simulink model "TITO_OCD_DE_2011"  (Simulink 7.7)
settings: Solver=ode4  SolverMode=SingleTasking  StartTime=0.0  StopTime=100  RelTol=1e-3  AbsTol=1e-6
libraries: simulink x40, stcsl_std x2
settings Model: Creator=chalupa  LastModifiedBy=NICHOLAS ANG
settings DataIOCC: LimitDataPoints=off  SignalLoggingSaveFormat=Dataset  SaveOutput=off  SaveTime=off
settings OptimizationCC: BlockReduction=off  BooleanDataType=off  ExpressionDepthLimit=128  InitFltsAndDblsToZero=on
settings DebuggingCC: SaveWithParameterizedLinksMsg=none  SignalResolutionControl=TryResolveAllWithWarning  SolverPrmCheckMsg=none  MultiTaskDSMMsg=warning  MultiTaskCondExecSysMsg=none  FcnCallInpInsideContextMsg=Enable All  StateNameClashWarn=none
settings HardwareCC: ProdBitPerPointer=64  ProdLargestAtomicFloat=Float  ProdIntDivRoundTo=Zero  ProdEndianess=LittleEndian  ProdHWDeviceType=Specified  TargetUnknown=on
settings RTWCC: TemplateMakefile=grt_msvc.tmf
settings CodeAppCC: CustomSymbolStrType=$N$R$M_T
settings GRTTargetCC: TargetFcnLib=ansi_tfl_tmw.mat  TargetFunctionLibrary=C89/C90 (ANSI)  GeneratePreprocessorConditionals=Use local settings

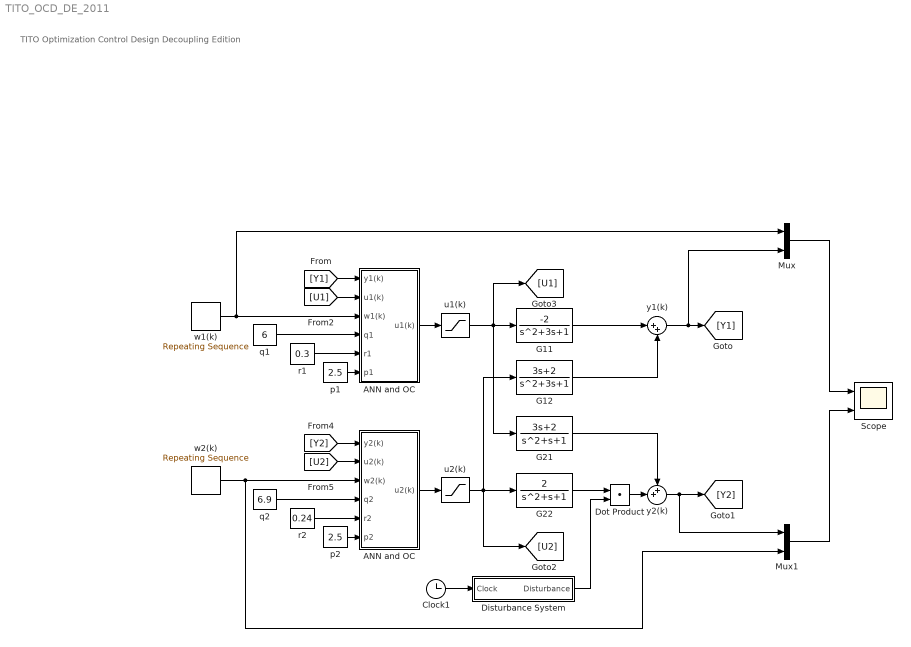
== system TITO_OCD_DE_2011 ==
  note: TITO Optimization Control Design Decoupling Edition
  " ANN and OC " : Subsystem
  ANN and OC : Subsystem
  Clock1 : Clock
  Disturbance System : Subsystem
  Dot Product : DotProduct  InputSameDT=on  OutDataTypeStr=Inherit: Inherit via internal rule
  G11 : TransferFcn  Numerator=[-2]  Denominator=[1 3 1]
  G12 : TransferFcn  Numerator=[3 2]  Denominator=[1 3 1]
  G21 : TransferFcn  Numerator=[3 2]  Denominator=[1 1 1]
  G22 : TransferFcn  Numerator=[2]  Denominator=[1 1 1]
  Mux : Mux  Inputs=2
  Mux1 : Mux  Inputs=2
  "Scope  " : Scope  NumInputPorts=2
      settings: TimeRange=auto  MaxDataPoints=5000  SaveToWorkspace=off  SaveName=ScopeData2  YMin=-1.079~-5  YMax=2.42451~5  SampleTime=-1
  p1 : Constant  Value=2.5
  p2 : Constant  Value=2.5
  q1 : Constant  Value=6
  q2 : Constant  Value=6.9
  r1 : Constant  Value=0.3
  r2 : Constant  Value=0.24
  u1(k) : Saturate  UpperLimit=1  LowerLimit=-1
  u2(k) : Saturate  UpperLimit=1  LowerLimit=-1
  w1(k) : simulink/Sources/Repeating Sequence  rep_seq_t=20*[0 0.4999 0.5 1.4999]  rep_seq_y=[1 1 2 2]
  w2(k) : simulink/Sources/Repeating Sequence  rep_seq_t=20*[0 0.9999 1.0 1.4999]  rep_seq_y=0.52*[1 1 2 2]
  y1(k) : Sum  Inputs=|++
  y2(k) : Sum  Inputs=++|
  wires:
  G11/1 -> y1(k)/1
  G21/1 -> y2(k)/1
  q1/1 -> ANN and OC/4(q1)
  r1/1 -> ANN and OC/5(r1)
  p1/1 -> ANN and OC/6(p1)
  q2/1 -> " ANN and OC "/4(q2)
  r2/1 -> " ANN and OC "/5(r2)
  p2/1 -> " ANN and OC "/6(p2)
  w1(k)/1 -> Mux/1, ANN and OC/3(w1(k))
  w2(k)/1 -> Mux1/2, " ANN and OC "/3(w2(k))
  y2(k)/1 -> Mux1/1, [Y2]
  G12/1 -> y1(k)/2
  [Y1] -> ANN and OC/1(y1(k))
  [U1] -> ANN and OC/2(u1(k))
  " ANN and OC "/1(" u2(k)") -> u2(k)/1
  [U2] -> " ANN and OC "/2(u2(k))
  [Y2] -> " ANN and OC "/1(y2(k))
  ANN and OC/1(" u1(k)") -> u1(k)/1
  u1(k)/1 -> [U1], G21/1, G11/1
  u2(k)/1 -> [U2], G12/1, G22/1
  Clock1/1 -> Disturbance System/1(Clock)
  G22/1 -> Dot Product/1
  Disturbance System/1(Disturbance) -> Dot Product/2
  Dot Product/1 -> y2(k)/2
  Mux/1 -> "Scope  "/1
  Mux1/1 -> "Scope  "/2
  y1(k)/1 -> Mux/2, [Y1]

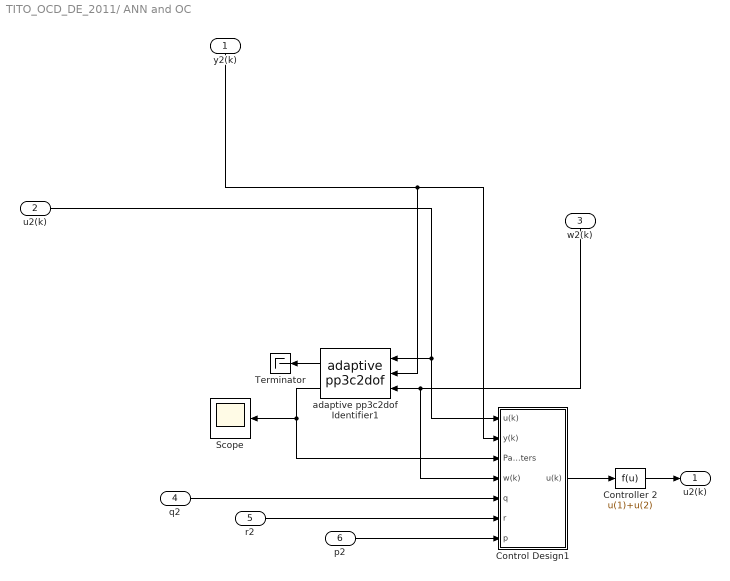
== system TITO_OCD_DE_2011/ ANN and OC  ==
  y2(k) : Inport
  u2(k) : Inport  Port=2
  w2(k) : Inport  Port=3
  q2 : Inport  Port=4
  r2 : Inport  Port=5
  p2 : Inport  Port=6
  " Controller 2 " : Fcn  Expr=u(1)+u(2)
  Control Design1 : Subsystem
  "Scope  " : Scope
      settings: TimeRange=auto  MaxDataPoints=5000  SaveToWorkspace=off  SaveName=ScopeData2  YMin=-1.20758  YMax=0.87657  SampleTime=-1
  Terminator : Terminator
  adaptive pp3c2dof Identifier1 : stcsl_std/Other simple adaptive controllers  using 3rd order models (3)/adaptive pp3c2dof  T0=0.1  ID_type=Least squares method (LSM)  Theta0=[0.1;0.2;0.3;0.4;0.5;0.6]  C0=1e9*eye(6)  phi0=1  lambda0=0.001  rho=0.99  nu0=1e-6  xi=1  omega=1
  " u2(k)" : Outport
  wires:
  y2(k)/1 -> Control Design1/2("y(k)  "), adaptive pp3c2dof Identifier1/2
  u2(k)/1 -> Control Design1/1("u(k)  "), adaptive pp3c2dof Identifier1/1
  adaptive pp3c2dof Identifier1/2 -> "Scope  "/1, Control Design1/3(Parameters)
  p2/1 -> Control Design1/7(p)
  r2/1 -> Control Design1/6(r)
  q2/1 -> Control Design1/5(q)
  Control Design1/1("u(k) ") -> " Controller 2 "/1
  w2(k)/1 -> Control Design1/4(w(k)), adaptive pp3c2dof Identifier1/3
  adaptive pp3c2dof Identifier1/1 -> Terminator/1
  " Controller 2 "/1 -> " u2(k)"/1

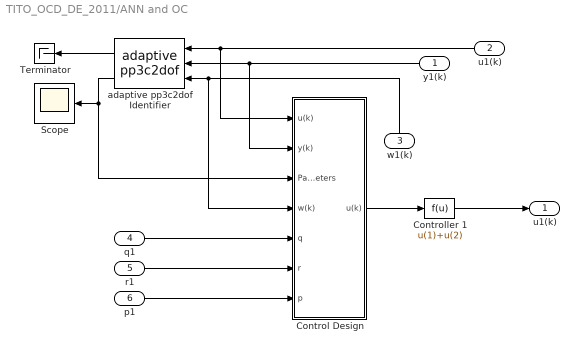
== system TITO_OCD_DE_2011/ANN and OC ==
  y1(k) : Inport
  u1(k) : Inport  Port=2
  w1(k) : Inport  Port=3
  q1 : Inport  Port=4
  r1 : Inport  Port=5
  p1 : Inport  Port=6
  " Controller 1 " : Fcn  Expr=u(1)+u(2)
  Control Design : Subsystem
  "Scope  " : Scope
      settings: TimeRange=auto  MaxDataPoints=5000  SaveToWorkspace=off  YMin=-0.80778  YMax=1.95673  SampleTime=-1
  Terminator : Terminator
  adaptive pp3c2dof Identifier : stcsl_std/Other simple adaptive controllers  using 3rd order models (3)/adaptive pp3c2dof  T0=0.1  ID_type=Least squares method (LSM)  Theta0=[0.1;0.2;0.3;0.4;0.5;0.6]  C0=1e9*eye(6)  phi0=1  lambda0=0.001  rho=0.99  nu0=1e-6  xi=1  omega=1
  " u1(k)" : Outport
  wires:
  u1(k)/1 -> Control Design/1("u(k)  "), adaptive pp3c2dof Identifier/1
  y1(k)/1 -> Control Design/2("y(k)  "), adaptive pp3c2dof Identifier/2
  adaptive pp3c2dof Identifier/2 -> "Scope  "/1, Control Design/3(Parameters)
  p1/1 -> Control Design/7(p)
  q1/1 -> Control Design/5(q)
  r1/1 -> Control Design/6(r)
  w1(k)/1 -> Control Design/4(w(k)), adaptive pp3c2dof Identifier/3
  adaptive pp3c2dof Identifier/1 -> Terminator/1
  Control Design/1("u(k) ") -> " Controller 1 "/1
  " Controller 1 "/1 -> " u1(k)"/1

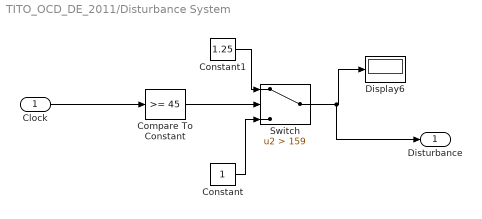
== system TITO_OCD_DE_2011/Disturbance System ==
  Clock : Inport
  Compare To Constant : simulink/Logic and Bit Operations/Compare To Constant  relop=>=  const=45  LogicOutDataTypeMode=boolean
  Constant : Constant
  Constant1 : Constant  Value=1.25
  Display6 : Display
  Switch : Switch  Criteria=u2 > Threshold  Threshold=159
  Disturbance : Outport
  wires:
  Compare To Constant/1 -> Switch/2
  Constant/1 -> Switch/3
  Constant1/1 -> Switch/1
  Switch/1 -> Disturbance/1, Display6/1
  Clock/1 -> Compare To Constant/1

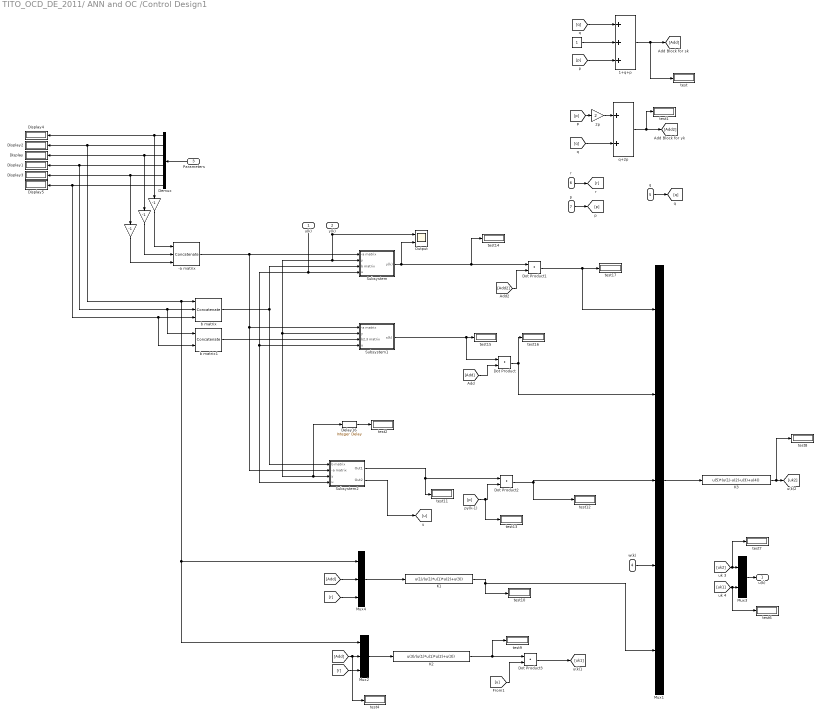
== system TITO_OCD_DE_2011/ ANN and OC /Control Design1 ==
  "u(k)  " : Inport
  "y(k)  " : Inport  Port=2
  Parameters : Inport  Port=3
  w(k) : Inport  Port=4
  q : Inport  Port=5
  r : Inport  Port=6
  p : Inport  Port=7
  " " : Gain  Gain=-1
  "   " : Gain  Gain=-1
  "    " : Gain  Gain=-1
  "      " : Constant
  -a matrix : Concatenate  NumInputs=3  Mode=Multidimensional array  ConcatenateDimension=2
  1+q+p : Sum  Inputs=+++
  2p : Gain  Gain=2
  Delay16 : simulink/Discrete/Integer Delay  NumDelays=1  vinit=0.0  samptime=-1
  Demux : Demux  Outputs=6
  Display{,1..5} (6 alike) : Display
  Dot Product{,1..3} (4 alike) : DotProduct  InputSameDT=on  OutDataTypeStr=Inherit: Inherit via internal rule
  K1 : Fcn  Expr=u(1)/(u(1)*u(1)*u(2)+u(3))
  K2 : Fcn  Expr=u(3)/(u(1)*u(1)*u(2)+u(3))
  K3 : Fcn  Expr=u(5)*(u(1)-u(2)-u(3)+u(4))
  Mux1 : Mux  Inputs=5
  Mux2 : Mux  Inputs=3
  Mux3 : Mux  Inputs=2
  Mux4 : Mux  Inputs=3
  Output : Scope  NumInputPorts=2
      settings: TimeRange=auto  MaxDataPoints=5000  SaveName=ScopeData222  YMin=-1.36833~-5  YMax=12.31494~5  SampleTime=-1
  Subsystem : Subsystem
  Subsystem1 : Subsystem
  Subsystem2 : Subsystem
  b matrix : Concatenate  NumInputs=3  Mode=Multidimensional array  ConcatenateDimension=2
  b matrix1 : Concatenate  Mode=Multidimensional array  ConcatenateDimension=2
  q+2p : Sum
  test{,1..2,4,6..17} (16 alike) : Display
  "u(k) " : Outport
  wires:
  "   "/1 -> -a matrix/1
  "    "/1 -> -a matrix/2
  " "/1 -> -a matrix/3
  b matrix/1 -> Subsystem2/1(b matrix), Subsystem/3(b matrix)
  -a matrix/1 -> Subsystem2/2(-a matrix), Subsystem1/1(-a matrix), Subsystem/1(-a matrix)
  Demux/6 -> b matrix1/2, b matrix/3, Display5/1
  Demux/1 -> "   "/1, Display4/1
  Demux/4 -> b matrix1/1, b matrix/2, Display1/1
  "u(k)  "/1 -> Subsystem2/4(u), Subsystem1/4(u), Subsystem/4(u)
  Mux4/1 -> K1/1
  q/1 -> [q]
  p/1 -> [p]
  r/1 -> [r]
  [p] -> 1+q+p/3
  1+q+p/1 -> test/1, [Add]
  [Add] -> Dot Product/2
  Dot Product/1 -> Mux1/2, test16/1
  [q] -> q+2p/2
  [p] -> 2p/1
  2p/1 -> q+2p/1
  q+2p/1 -> test1/1, [Add2]
  [Add2] -> Dot Product1/2
  Dot Product1/1 -> Mux1/1, test17/1
  [p] -> test13/1, Dot Product2/2
  Dot Product2/1 -> test12/1, Mux1/3
  K1/1 -> test10/1, Mux1/5
  [r] -> Mux4/3
  [Add] -> Mux4/2
  Mux1/1 -> K3/1
  Mux2/1 -> K2/1
  [r] -> Mux2/3
  [Add] -> test4/1, Mux2/2
  K2/1 -> test9/1, Dot Product3/1
  [u] -> Dot Product3/2
  Dot Product3/1 -> [uk1]
  K3/1 -> test8/1, [uk2]
  Mux3/1 -> "u(k) "/1
  [uk2] -> test7/1, Mux3/1
  [uk1] -> test6/1, Mux3/2
  [q] -> 1+q+p/1
  "      "/1 -> 1+q+p/2
  Subsystem/1(y(k)) -> Dot Product1/1, test14/1, Output/2
  Subsystem1/1(s(k)) -> Dot Product/1, test15/1
  b matrix1/1 -> Subsystem1/3(b2,3 matrix)
  Subsystem2/1(Out1) -> test11/1, Dot Product2/1
  Subsystem2/2(Out2) -> [u]
  w(k)/1 -> Mux1/4
  Demux/2 -> Mux4/1, Mux2/1, b matrix/1, Display2/1
  Demux/5 -> Display3/1, " "/1
  Parameters/1 -> Demux/1
  Demux/3 -> "    "/1, Display/1
  "y(k)  "/1 -> Delay16/1, Subsystem2/3(y), Subsystem1/2(y), Subsystem/2(y), Output/1
  Delay16/1 -> test2/1

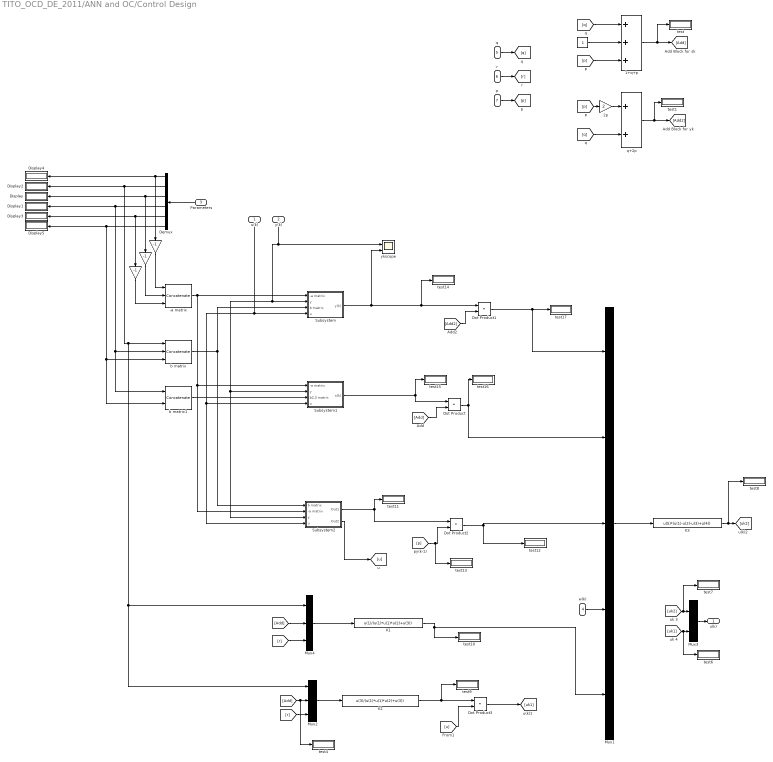
== system TITO_OCD_DE_2011/ANN and OC/Control Design ==
  "u(k)  " : Inport
  "y(k)  " : Inport  Port=2
  Parameters : Inport  Port=3
  w(k) : Inport  Port=4
  q : Inport  Port=5
  r : Inport  Port=6
  p : Inport  Port=7
  " " : Gain  Gain=-1
  "   " : Gain  Gain=-1
  "    " : Gain  Gain=-1
  "      " : Constant
  -a matrix : Concatenate  NumInputs=3  Mode=Multidimensional array  ConcatenateDimension=2
  1+q+p : Sum  Inputs=+++
  2p : Gain  Gain=2
  Demux : Demux  Outputs=6
  Display{,1..5} (6 alike) : Display
  Dot Product{,1..3} (4 alike) : DotProduct  InputSameDT=on  OutDataTypeStr=Inherit: Inherit via internal rule
  K1 : Fcn  Expr=u(1)/(u(1)*u(1)*u(2)+u(3))
  K2 : Fcn  Expr=u(3)/(u(1)*u(1)*u(2)+u(3))
  K3 : Fcn  Expr=u(5)*(u(1)-u(2)-u(3)+u(4))
  Mux1 : Mux  Inputs=5
  Mux2 : Mux  Inputs=3
  Mux3 : Mux  Inputs=2
  Mux4 : Mux  Inputs=3
  Subsystem : Subsystem
  Subsystem1 : Subsystem
  Subsystem2 : Subsystem
  b matrix : Concatenate  NumInputs=3  Mode=Multidimensional array  ConcatenateDimension=2
  b matrix1 : Concatenate  Mode=Multidimensional array  ConcatenateDimension=2
  q+2p : Sum
  test{,1,4,6..17} (15 alike) : Display
  ykscope : Scope  NumInputPorts=2
      settings: TimeRange=auto  MaxDataPoints=5000  SaveToWorkspace=off  YMin=-5.59859~-5  YMax=3.73184~5  SampleTime=-1
  "u(k) " : Outport
  wires:
  "   "/1 -> -a matrix/1
  "    "/1 -> -a matrix/2
  " "/1 -> -a matrix/3
  b matrix/1 -> Subsystem2/1(b matrix), Subsystem/3(b matrix)
  -a matrix/1 -> Subsystem2/2(-a matrix), Subsystem1/1(-a matrix), Subsystem/1(-a matrix)
  Demux/6 -> b matrix1/2, b matrix/3, Display5/1
  Demux/1 -> "   "/1, Display4/1
  Demux/4 -> b matrix1/1, b matrix/2, Display1/1
  "u(k)  "/1 -> Subsystem2/4(u), Subsystem1/4(u), Subsystem/4(u)
  "y(k)  "/1 -> Subsystem2/3(y), Subsystem1/2(y), Subsystem/2(y), ykscope/1
  Mux4/1 -> K1/1
  q/1 -> [q]
  p/1 -> [p]
  r/1 -> [r]
  [p] -> 1+q+p/3
  1+q+p/1 -> test/1, [Add]
  [Add] -> Dot Product/2
  Dot Product/1 -> Mux1/2, test16/1
  [q] -> q+2p/2
  [p] -> 2p/1
  2p/1 -> q+2p/1
  q+2p/1 -> test1/1, [Add2]
  [Add2] -> Dot Product1/2
  Dot Product1/1 -> Mux1/1, test17/1
  [p] -> test13/1, Dot Product2/2
  Dot Product2/1 -> test12/1, Mux1/3
  K1/1 -> test10/1, Mux1/5
  [r] -> Mux4/3
  [Add] -> Mux4/2
  Mux1/1 -> K3/1
  Mux2/1 -> K2/1
  [r] -> Mux2/3
  [Add] -> test4/1, Mux2/2
  K2/1 -> test9/1, Dot Product3/1
  [u] -> Dot Product3/2
  Dot Product3/1 -> [uk1]
  K3/1 -> test8/1, [uk2]
  Mux3/1 -> "u(k) "/1
  [uk2] -> test7/1, Mux3/1
  [uk1] -> test6/1, Mux3/2
  [q] -> 1+q+p/1
  "      "/1 -> 1+q+p/2
  Subsystem/1(y(k)) -> ykscope/2, Dot Product1/1, test14/1
  Subsystem1/1(s(k)) -> test15/1, Dot Product/1
  b matrix1/1 -> Subsystem1/3(b2,3 matrix)
  Subsystem2/1(Out1) -> Dot Product2/1, test11/1
  Subsystem2/2(Out2) -> [u]
  w(k)/1 -> Mux1/4
  Demux/2 -> Mux4/1, Mux2/1, b matrix/1, Display2/1
  Demux/5 -> Display3/1, " "/1
  Parameters/1 -> Demux/1
  Demux/3 -> "    "/1, Display/1

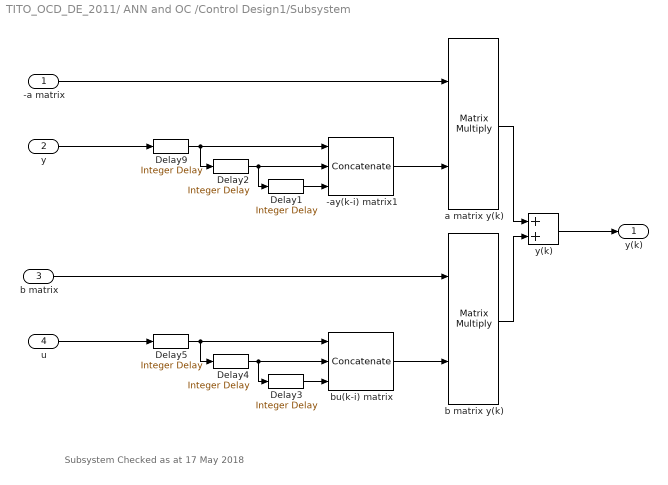
== system TITO_OCD_DE_2011/ ANN and OC /Control Design1/Subsystem ==
  note: Subsystem Checked as at 17 May 2018
  -a matrix : Inport
  y : Inport  Port=2
  b matrix : Inport  Port=3
  u : Inport  Port=4
  -ay(k-i) matrix1 : Concatenate  NumInputs=3  Mode=Multidimensional array
  Delay{1..5,9} (6 alike) : simulink/Discrete/Integer Delay  NumDelays=1  vinit=0.0  samptime=-1
  a matrix y(k) : Product  Multiplication=Matrix(*)
  b matrix y(k) : Product  Multiplication=Matrix(*)
  bu(k-i) matrix : Concatenate  NumInputs=3  Mode=Multidimensional array
  "y(k) " : Sum
  y(k) : Outport
  wires:
  "y(k) "/1 -> y(k)/1
  y/1 -> Delay9/1
  b matrix/1 -> b matrix y(k)/1
  -a matrix/1 -> a matrix y(k)/1
  u/1 -> Delay5/1
  b matrix y(k)/1 -> "y(k) "/2
  Delay9/1 -> Delay2/1, -ay(k-i) matrix1/1
  Delay1/1 -> -ay(k-i) matrix1/3
  Delay5/1 -> Delay4/1, bu(k-i) matrix/1
  Delay2/1 -> Delay1/1, -ay(k-i) matrix1/2
  bu(k-i) matrix/1 -> b matrix y(k)/2
  -ay(k-i) matrix1/1 -> a matrix y(k)/2
  Delay4/1 -> Delay3/1, bu(k-i) matrix/2
  a matrix y(k)/1 -> "y(k) "/1
  Delay3/1 -> bu(k-i) matrix/3

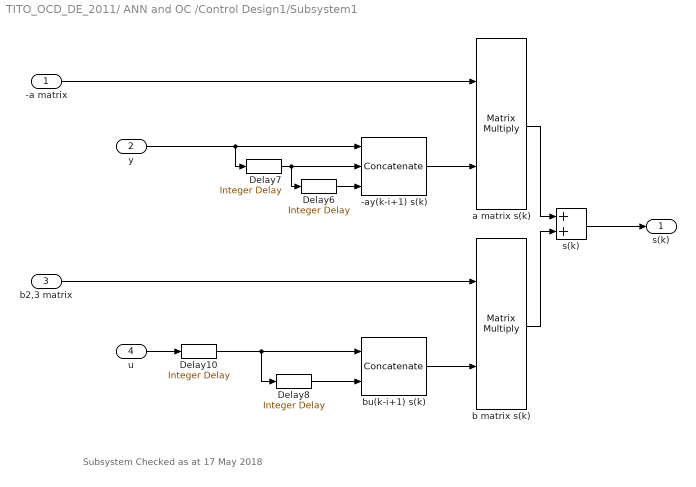
== system TITO_OCD_DE_2011/ ANN and OC /Control Design1/Subsystem1 ==
  note: Subsystem Checked as at 17 May 2018
  -a matrix : Inport
  y : Inport  Port=2
  b2,3 matrix : Inport  Port=3
  u : Inport  Port=4
  -ay(k-i+1) s(k) : Concatenate  NumInputs=3  Mode=Multidimensional array
  Delay{6..8,10} (4 alike) : simulink/Discrete/Integer Delay  NumDelays=1  vinit=0.0  samptime=-1
  a matrix s(k) : Product  Multiplication=Matrix(*)
  b matrix s(k) : Product  Multiplication=Matrix(*)
  "bu(k-i+1) s(k) " : Concatenate  Mode=Multidimensional array
  "s(k) " : Sum
  s(k) : Outport
  wires:
  "s(k) "/1 -> s(k)/1
  a matrix s(k)/1 -> "s(k) "/1
  b matrix s(k)/1 -> "s(k) "/2
  Delay6/1 -> -ay(k-i+1) s(k)/3
  "bu(k-i+1) s(k) "/1 -> b matrix s(k)/2
  Delay8/1 -> "bu(k-i+1) s(k) "/2
  b2,3 matrix/1 -> b matrix s(k)/1
  -ay(k-i+1) s(k)/1 -> a matrix s(k)/2
  Delay10/1 -> "bu(k-i+1) s(k) "/1, Delay8/1
  Delay7/1 -> Delay6/1, -ay(k-i+1) s(k)/2
  -a matrix/1 -> a matrix s(k)/1
  u/1 -> Delay10/1
  y/1 -> Delay7/1, -ay(k-i+1) s(k)/1

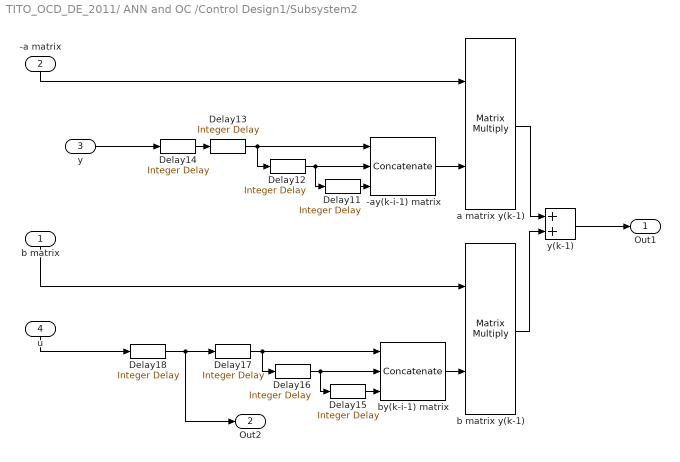
== system TITO_OCD_DE_2011/ ANN and OC /Control Design1/Subsystem2 ==
  b matrix : Inport
  -a matrix : Inport  Port=2
  y : Inport  Port=3
  u : Inport  Port=4
  -ay(k-i-1) matrix : Concatenate  NumInputs=3  Mode=Multidimensional array
  Delay{11..18} (8 alike) : simulink/Discrete/Integer Delay  NumDelays=1  vinit=0.0  samptime=-1
  a matrix y(k-1) : Product  Multiplication=Matrix(*)
  b matrix y(k-1) : Product  Multiplication=Matrix(*)
  by(k-i-1) matrix : Concatenate  NumInputs=3  Mode=Multidimensional array
  y(k-1) : Sum
  Out1 : Outport
  Out2 : Outport  Port=2
  wires:
  y(k-1)/1 -> Out1/1
  b matrix y(k-1)/1 -> y(k-1)/2
  Delay14/1 -> Delay13/1
  Delay18/1 -> Out2/1, Delay17/1
  Delay15/1 -> by(k-i-1) matrix/3
  Delay16/1 -> Delay15/1, by(k-i-1) matrix/2
  Delay17/1 -> by(k-i-1) matrix/1, Delay16/1
  Delay12/1 -> Delay11/1, -ay(k-i-1) matrix/2
  Delay13/1 -> -ay(k-i-1) matrix/1, Delay12/1
  Delay11/1 -> -ay(k-i-1) matrix/3
  -a matrix/1 -> a matrix y(k-1)/1
  y/1 -> Delay14/1
  u/1 -> Delay18/1
  b matrix/1 -> b matrix y(k-1)/1
  a matrix y(k-1)/1 -> y(k-1)/1
  by(k-i-1) matrix/1 -> b matrix y(k-1)/2
  -ay(k-i-1) matrix/1 -> a matrix y(k-1)/2

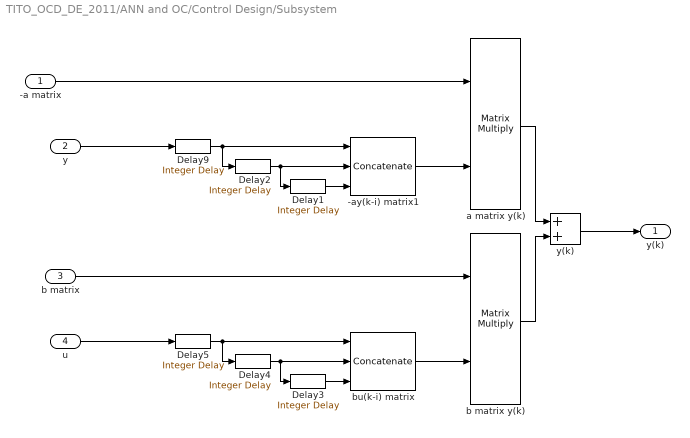
== system TITO_OCD_DE_2011/ANN and OC/Control Design/Subsystem ==
  -a matrix : Inport
  y : Inport  Port=2
  b matrix : Inport  Port=3
  u : Inport  Port=4
  -ay(k-i) matrix1 : Concatenate  NumInputs=3  Mode=Multidimensional array
  Delay{1..5,9} (6 alike) : simulink/Discrete/Integer Delay  NumDelays=1  vinit=0.0  samptime=-1
  a matrix y(k) : Product  Multiplication=Matrix(*)
  b matrix y(k) : Product  Multiplication=Matrix(*)
  bu(k-i) matrix : Concatenate  NumInputs=3  Mode=Multidimensional array
  "y(k) " : Sum
  y(k) : Outport
  wires:
  "y(k) "/1 -> y(k)/1
  y/1 -> Delay9/1
  b matrix/1 -> b matrix y(k)/1
  -a matrix/1 -> a matrix y(k)/1
  u/1 -> Delay5/1
  b matrix y(k)/1 -> "y(k) "/2
  Delay9/1 -> Delay2/1, -ay(k-i) matrix1/1
  Delay1/1 -> -ay(k-i) matrix1/3
  Delay5/1 -> Delay4/1, bu(k-i) matrix/1
  Delay2/1 -> Delay1/1, -ay(k-i) matrix1/2
  bu(k-i) matrix/1 -> b matrix y(k)/2
  -ay(k-i) matrix1/1 -> a matrix y(k)/2
  Delay4/1 -> Delay3/1, bu(k-i) matrix/2
  a matrix y(k)/1 -> "y(k) "/1
  Delay3/1 -> bu(k-i) matrix/3

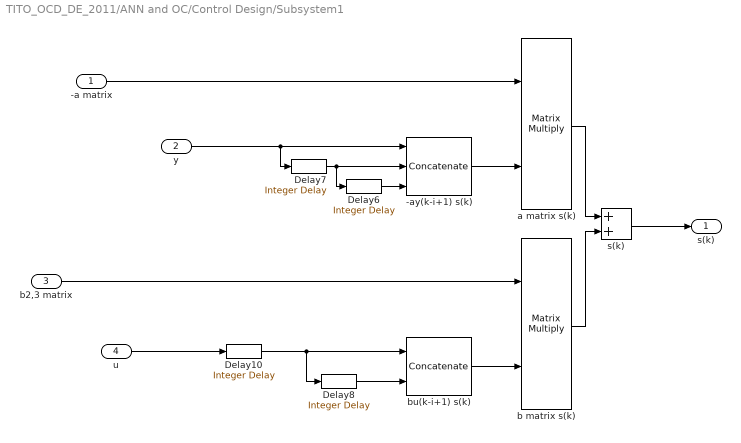
== system TITO_OCD_DE_2011/ANN and OC/Control Design/Subsystem1 ==
  -a matrix : Inport
  y : Inport  Port=2
  b2,3 matrix : Inport  Port=3
  u : Inport  Port=4
  -ay(k-i+1) s(k) : Concatenate  NumInputs=3  Mode=Multidimensional array
  Delay{6..8,10} (4 alike) : simulink/Discrete/Integer Delay  NumDelays=1  vinit=0.0  samptime=-1
  a matrix s(k) : Product  Multiplication=Matrix(*)
  b matrix s(k) : Product  Multiplication=Matrix(*)
  "bu(k-i+1) s(k) " : Concatenate  Mode=Multidimensional array
  "s(k) " : Sum
  s(k) : Outport
  wires:
  "s(k) "/1 -> s(k)/1
  a matrix s(k)/1 -> "s(k) "/1
  b matrix s(k)/1 -> "s(k) "/2
  Delay6/1 -> -ay(k-i+1) s(k)/3
  "bu(k-i+1) s(k) "/1 -> b matrix s(k)/2
  Delay8/1 -> "bu(k-i+1) s(k) "/2
  b2,3 matrix/1 -> b matrix s(k)/1
  -ay(k-i+1) s(k)/1 -> a matrix s(k)/2
  Delay10/1 -> "bu(k-i+1) s(k) "/1, Delay8/1
  Delay7/1 -> Delay6/1, -ay(k-i+1) s(k)/2
  -a matrix/1 -> a matrix s(k)/1
  u/1 -> Delay10/1
  y/1 -> Delay7/1, -ay(k-i+1) s(k)/1

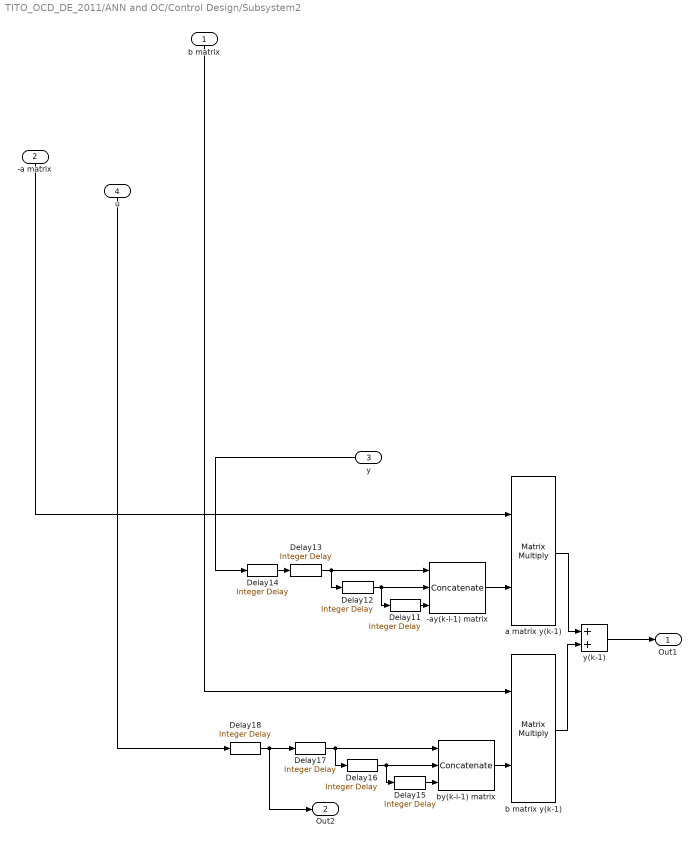
== system TITO_OCD_DE_2011/ANN and OC/Control Design/Subsystem2 ==
  b matrix : Inport
  -a matrix : Inport  Port=2
  y : Inport  Port=3
  u : Inport  Port=4
  -ay(k-i-1) matrix : Concatenate  NumInputs=3  Mode=Multidimensional array
  Delay{11..18} (8 alike) : simulink/Discrete/Integer Delay  NumDelays=1  vinit=0.0  samptime=-1
  a matrix y(k-1) : Product  Multiplication=Matrix(*)
  b matrix y(k-1) : Product  Multiplication=Matrix(*)
  by(k-i-1) matrix : Concatenate  NumInputs=3  Mode=Multidimensional array
  y(k-1) : Sum
  Out1 : Outport
  Out2 : Outport  Port=2
  wires:
  y(k-1)/1 -> Out1/1
  b matrix y(k-1)/1 -> y(k-1)/2
  Delay14/1 -> Delay13/1
  Delay18/1 -> Out2/1, Delay17/1
  Delay15/1 -> by(k-i-1) matrix/3
  Delay16/1 -> Delay15/1, by(k-i-1) matrix/2
  Delay17/1 -> by(k-i-1) matrix/1, Delay16/1
  Delay12/1 -> Delay11/1, -ay(k-i-1) matrix/2
  Delay13/1 -> -ay(k-i-1) matrix/1, Delay12/1
  Delay11/1 -> -ay(k-i-1) matrix/3
  -a matrix/1 -> a matrix y(k-1)/1
  y/1 -> Delay14/1
  u/1 -> Delay18/1
  b matrix/1 -> b matrix y(k-1)/1
  a matrix y(k-1)/1 -> y(k-1)/1
  by(k-i-1) matrix/1 -> b matrix y(k-1)/2
  -ay(k-i-1) matrix/1 -> a matrix y(k-1)/2
